simulink model "segway_sm"  (R2023b)
settings: Solver=VariableStepAuto  StartTime=0.0  StopTime=100  RelTol=1e-3
values from neighbouring files (symbols this model uses):
  probni1 = preko_funkcije_acker(1)    [segway.m]
  probni2 = preko_funkcije_acker(2)    [segway.m]
  probni3 = preko_funkcije_acker(3)    [segway.m]
  probni4 = preko_funkcije_acker(4)    [segway.m]
libraries: cstblocks x1
settings Model: Creator=HP  LastModifiedBy=HP

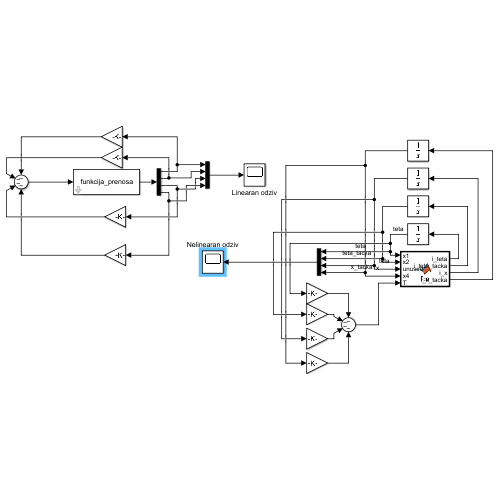
[thumbnail: Simulink's stored preview of the top-level diagram]
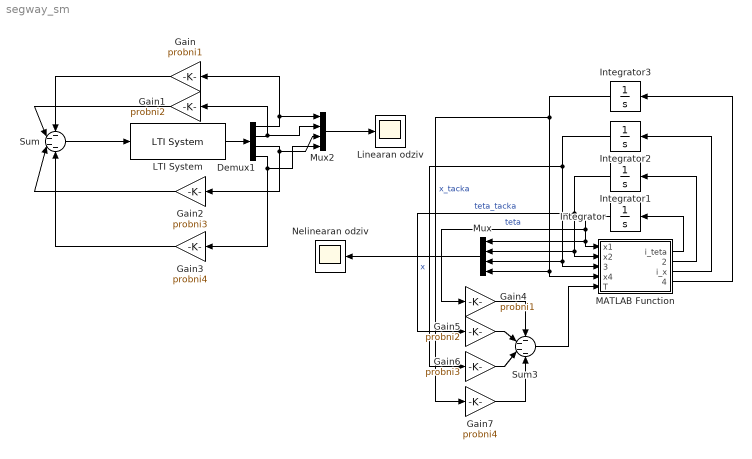
== system segway_sm ==
  Demux1 : Demux
  Gain : Gain  Gain=probni1
  Gain1 : Gain  Gain=probni2
  Gain2 : Gain  Gain=probni3
  Gain3 : Gain  Gain=probni4
  Gain4 : Gain  Gain=probni1
  Gain5 : Gain  Gain=probni2
  Gain6 : Gain  Gain=probni3
  Gain7 : Gain  Gain=probni4
  Integrator{,1..3} (4 alike) : Integrator
  LTI System : cstblocks/LTI System  sys=funkcija_prenosa  IC=[]  PadeOrder=0
  Linearan odziv : Scope
  MATLAB Function : MATLAB Function  TreatAsAtomicUnit=on
  Mux : Mux
  Mux2 : Mux
  Nelinearan odziv : Scope
  Sum : Sum  Inputs=----
  Sum3 : Sum  Inputs=----
  wires:
  MATLAB Function/1(i_teta) -> Integrator/1
  MATLAB Function/2(i_teta_tacka) -> Integrator1/1
  MATLAB Function/3(i_x) -> Integrator2/1
  MATLAB Function/4(i_x_tacka) -> Integrator3/1
  Integrator1/1 -> Gain5/1, MATLAB Function/2(x2), Mux/2  "teta_tacka"
  Integrator2/1 -> Gain6/1, MATLAB Function/3(unused), Mux/3  "x"
  Integrator3/1 -> Gain7/1, MATLAB Function/4(x4), Mux/4  "x_tacka"
  Mux/1 -> Nelinearan odziv/1
  LTI System/1 -> Demux1/1
  Demux1/1 -> Mux2/1, Gain/1
  Demux1/2 -> Mux2/2, Gain1/1
  Demux1/3 -> Mux2/3, Gain2/1
  Demux1/4 -> Mux2/4, Gain3/1
  Sum/1 -> LTI System/1
  Gain1/1 -> Sum/2
  Gain2/1 -> Sum/3
  Gain3/1 -> Sum/4
  Mux2/1 -> Linearan odziv/1
  Gain4/1 -> Sum3/1
  Gain5/1 -> Sum3/2
  Gain6/1 -> Sum3/3
  Gain7/1 -> Sum3/4
  Sum3/1 -> MATLAB Function/5(T)
  Integrator/1 -> Gain4/1, MATLAB Function/1(x1), Mux/1  "teta"
  Gain/1 -> Sum/1

== matlab function segway_sm/MATLAB Function ==
  data: x1 input size=1; x2 input size=1; unused input; x4 input size=1; i_teta output size=1; i_teta_tacka output size=1; i_x output size=1; i_x_tacka output size=1; T input size=1
function [i_teta, i_teta_tacka, i_x, i_x_tacka] = fcn(x1, x2, ~, x4, T)

m = 85; 
M = 3.5; 
l = 1.7; 
g = 9.81;
R = 0.05; 
Iw = 0.07; 
Ir = 68.98; 
K = 1;
k1 = (M + m) * R + Iw/R;
k2 = m*l*R;
k3 = m*l;
k4 = Ir + m*l*l;
k5 = m*l*g;
k6 = m*l*R;

% if T == 1
%     x1 = 0.00003; 
%     x2 = 0; %teta
%     %x3 = 0;
%     x4 = 0;
% end

i_teta = x2;
i_teta_tacka = ((T + k6 * sin(x1) * x2 * x2 -    (k1  * k5 * sin(x1)  - K * T * k1)   /  (k3*cos(x1))) /(k2*cos(x1) - (k1*k4)/(k3*cos(x1))));
i_x = x4;
i_x_tacka = ((k5*sin(x1) - K * T - k4 *  ((T + k6 * sin(x1) * x2 * x2 -    (k1 * k5 * sin(x1)  - K * T * k1)   /  (k3*cos(x1))) /(k2*cos(x1) - k1*k4/(k3*cos(x1)))))/(k3*cos(x1)));
